simulink model "zad1_4"  (R2019b)
settings: Solver=ode4  StartTime=0.0  StopTime=5  FixedStep=0.000001  MaxStep=10e-6  RelTol=1e-3
values from neighbouring files (symbols this model uses):
  C = 0.000001    (= 1e-06)    [skr_1_4.m]    (also in skrypt_1_4.m = 0.1; skrypt_1_4_1.m = vC(z))
  R = 1000000    [skr_1_4.m]    (also in skrypt_1_4.m = 100; skrypt_1_4_1.m = 10)
settings Model: Creator=marci  LastModifiedBy=marci

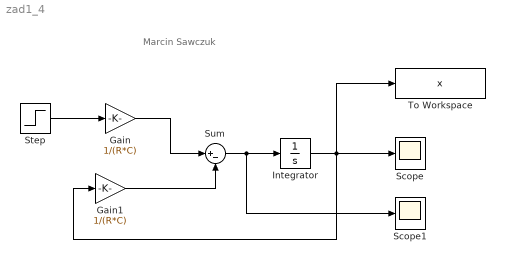
== system zad1_4 ==
  note: Marcin Sawczuk
  Gain : Gain  Gain=1/(R*C)
  Gain1 : Gain  Gain=1/(R*C)
  Integrator : Integrator  InitialCondition=-1.72
  Scope : Scope
  Scope1 : Scope
  Step : Step  Before=1  After=0  SampleTime=0
  Sum : Sum  Inputs=|+-
  To Workspace : ToWorkspace  VariableName=x  SaveFormat=Timeseries  SampleTime=-1
  wires:
  Gain/1 -> Sum/1
  Sum/1 -> Scope1/1, Integrator/1
  Gain1/1 -> Sum/2
  Step/1 -> Gain/1
  Integrator/1 -> Gain1/1, To Workspace/1, Scope/1
